simulink model "Gen2"  (R2018b)
settings: Solver=VariableStepAuto  StartTime=0.0  StopTime=0.35  RelTol=1e-3
libraries: powerlib_meascontrol x1, powerlib x1
settings Model: Creator=User  LastModifiedBy=User
settings DataIOCC: ReturnWorkspaceOutputs=on
settings DebuggingCC: UnconnectedInputMsg=none  UnconnectedOutputMsg=none  UnconnectedLineMsg=none
settings ModelReferenceCC: EnableRefExpFcnMdlSchedulingChecks=off
settings RTWCC: Description=Generic Real-Time Target

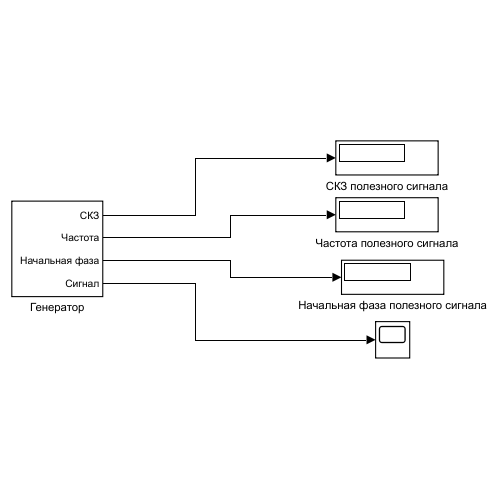
[thumbnail: Simulink's stored preview of the top-level diagram]
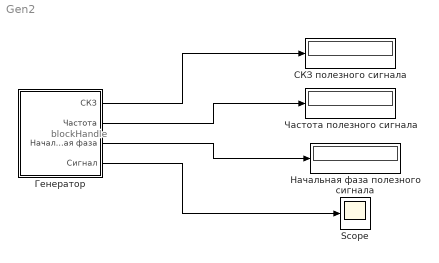
== system Gen2 ==
  note: blockHandle
  Scope : Scope
  Генератор : Subsystem  mask{flik_en=off, Ufl=0.25, Ffl=10, afl=0, fliker_on=1, noise_en=off, n_min_v=0, n_max_v=1, noise_on=1, U=1, F=50, a=0, Const=0}
      mask prompts: flik_en "Включить"; Ufl "Амплитуда(В)"; Ffl "Частота(Гц)"; afl "Начальная фаза(Рад)"; fliker_on "Включение фликера с помощью ключа"; noise_en "Включить"; n_min_v "Минимальное значение(В)"; n_max_v "Максимальное значение(В)"; noise_on "Вкючение шума с помощью ключа"; U "Амплитуда(В)"; F "Частота(Гц)"; a "Начальная фаза(Рад)"; Const "Постоянная составляющая(В)"
      mask DialogControl ParameterGroupVar Prompt: Параметр генератора
      mask DialogControl flik_params Prompt: Фликер
      mask DialogControl noise_params Prompt: Шум
      mask DialogControl Container5 Prompt: Полезный сигнал
  Начальная фаза полезного сигнала : Display
  СКЗ полезного сигнала : Display
  Частота полезного сигнала : Display
  wires:
  Генератор/1(СКЗ) -> СКЗ полезного сигнала/1
  Генератор/2(Частота) -> Частота полезного сигнала/1
  Генератор/3(Начальная фаза) -> Начальная фаза полезного сигнала/1
  Генератор/4(Сигнал) -> Scope/1

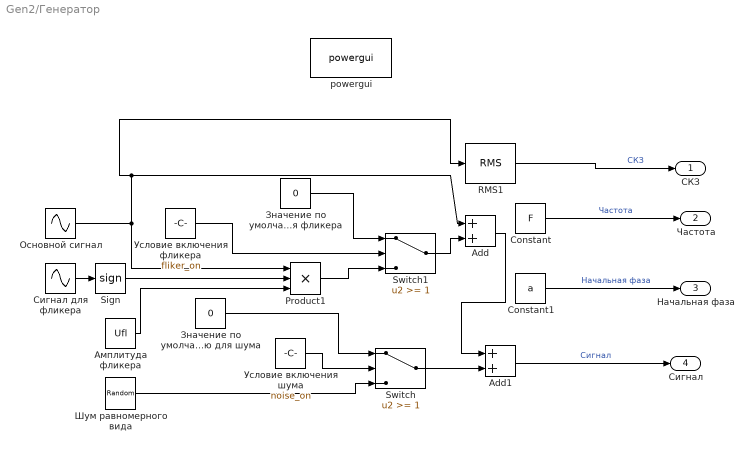
== system Gen2/Генератор ==
  Add : Sum
  Add1 : Sum
  Constant : Constant  Value=F
  Constant1 : Constant  Value=a
  Product1 : Product  Inputs=3
  RMS1 : powerlib_meascontrol/Measurements/RMS  TrueRMS=on  Freq=50  RMSInit=0  Ts=0
  Sign : Signum
  Switch : Switch  Threshold=1
  Switch1 : Switch  Threshold=1
  powergui : powerlib/powergui  Priority=1  SimulationMode=Continuous  SampleTime=50e-6  frequency=60  Iterations=50  frequencyindice=60  Pbase=100e6  ErrMax=1e-4  UnitsV=kV  UnitsW=MW  buscounter=0  FunctionMessages=off  echomessages=off  EnableUseOfTLC=off  CurrentSourceSwitches=off  DisableSnubberDevices=off  DisableRonSwitches=off  DisableVfSwitches=off  DisplayEquations=off  AutomaticDiscreteSolvers=off  SolverType=Tustin/Backward Euler (TBE)  Interpol=off  ExternalGateDelay=off  methode=off  Ts=100  x0status=blocks  SPID=on  SwTol=0  HookPort=off  NonlinearTolerance=1e-4  nMaxIteration=100  ContinueOnMaxIteration=off  RestoreLinks=warning  ResistiveCurrentMeasurement=off  Frange=[0:2:500]  Ylog=off  Xlog=on  ShowGrid=off  save=off  variable=ZData  structure=0  ZoomFFT=off  StartTime=0.0  cycles=1  DisplayStyle=1  fundamental=60  FreqAxis=off  MaxFrequency=1000  frequencyindicesteady=1  RmsSteady=1  display=off
  Амплитуда фликера : Constant  Value=Ufl  VectorParams1D=off
  Значение по умолчанию для шума : Constant  Value=0
  Значение по умолчанию для фликера : Constant  Value=0
  Основной сигнал : Sin  Amplitude=U  Bias=Const  Frequency=2*pi*F  Phase=a  SampleTime=0.000001
  Сигнал для фликера : Sin  Frequency=2*pi*Ffl  Phase=afl  SampleTime=0.000001
  Условие включения фликера : Constant  Value=fliker_on
  Условие включения шума : Constant  Value=noise_on  VectorParams1D=off
  Шум равномерного вида : UniformRandomNumber  Minimum=n_min_v  Maximum=n_max_v  SampleTime=0.0001
  СКЗ : Outport
  Частота : Outport  Port=2
  Начальная фаза : Outport  Port=3
  Сигнал : Outport  Port=4
  wires:
  Значение по умолчанию для шума/1 -> Switch/1
  Switch1/1 -> Add/2
  Switch/1 -> Add1/2
  Амплитуда фликера/1 -> Product1/3
  Product1/1 -> Switch1/3
  Add/1 -> Add1/1
  Add1/1 -> Сигнал/1  "Сигнал"
  Основной сигнал/1 -> Add/1, RMS1/1, Product1/1
  Сигнал для фликера/1 -> Sign/1
  Шум равномерного вида/1 -> Switch/3
  Sign/1 -> Product1/2
  RMS1/1 -> СКЗ/1  "СКЗ"
  Constant1/1 -> Начальная фаза/1  "Начальная фаза"
  Constant/1 -> Частота/1  "Частота"
  Условие включения шума/1 -> Switch/2
  Значение по умолчанию для фликера/1 -> Switch1/1
  Условие включения фликера/1 -> Switch1/2
